simulink model "ARDroneReplay_V2_second"  (R2020a)
settings: Solver=ode1  StartTime=0.0  StopTime=30  FixedStep=sampleTime  RelTol=1e-3  EnableMultiTasking=on
undefined symbols (not defined in the file): Continuous, sampleTime, Time
libraries: ctrlSharedLib x2, ARBlocks x1
settings Model: SimulationMode=accelerator  ExtModeTrigDuration=100000  Creator=Paul  LastModifiedBy=TowerWindows
settings DataIOCC: LimitDataPoints=on  SaveFormat=Array  SignalLoggingSaveFormat=ModelDataLogs  ReturnWorkspaceOutputs=off  TimeSaveName=time
settings OptimizationCC: ExpressionDepthLimit=2147483647  InitFltsAndDblsToZero=on
settings DebuggingCC: UnderspecifiedInitializationDetection=Classic  MergeDetectMultiDrivingBlocksExec=none  SolverPrmCheckMsg=warning  FcnCallInpInsideContextMsg=warning  StateNameClashWarn=warning  SFUnexpectedBacktrackingDiag=warning  SFNoUnconditionalDefaultTransitionDiag=warning  SFExecutionAtInitializationDiag=none  ArithmeticOperatorsInVariantConditions=warning
settings ModelReferenceCC: PropagateSignalLabelsOutOfModel=off
settings SFSimCC: SimUseLocalCustomCode=off  CustomCodeUndefinedFunction=UseInterfaceOnly
settings RTWCC: Description=Simulink Desktop Real-Time  SystemTargetFile=sldrt.tlc  TemplateMakefile=sldrt.tmf  RTWUseLocalCustomCode=off  RTWCompilerOptimization=on
settings CodeAppCC: MaxIdLength=95  StateflowObjectComments=on
settings SimulinkDesktopRealTimeCC: TargetPreCompLibLocation=C:\Program Files\MATLAB\R2020a\toolbox\sldrt\lib\win64  TargetLangStandard=C89/C90 (ANSI)  SupportVariableSizeSignals=off
settings ConfigComp: CovMetricSettings=dw  CovHtmlReporting=on  CovSaveCumulativeToWorkspaceVar=on  CovSaveSingleToWorkspaceVar=on  CovExternalEMLEnable=off

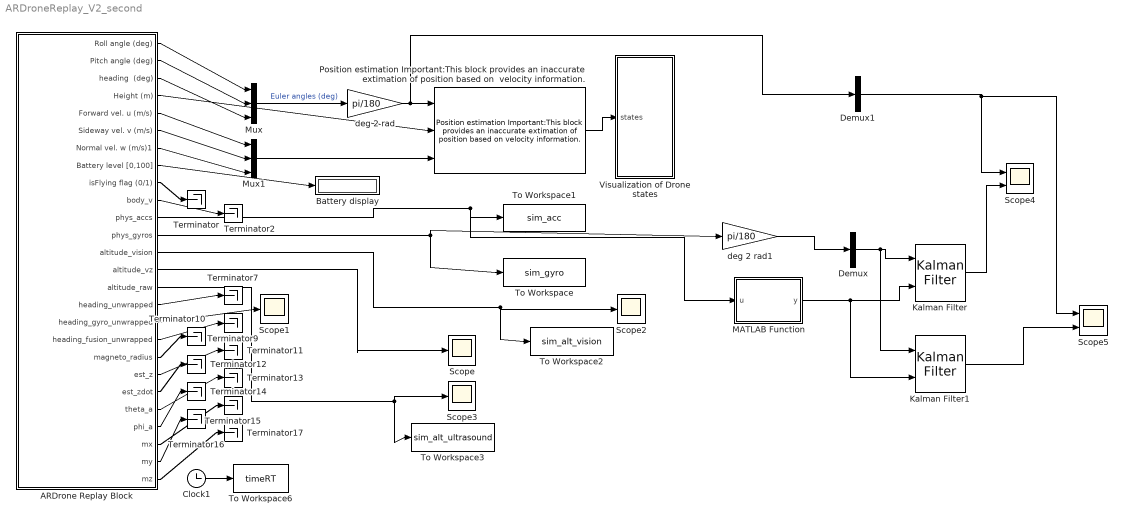
== system ARDroneReplay_V2_second ==
  ARDrone Replay Block : Subsystem  AncestorBlock="ARBlocks/ARDrone Wi-Fi  Block"
  Battery display : Display
  Clock1 : Clock
  Demux : Demux  Outputs=3
  Demux1 : Demux  Outputs=3
  Kalman Filter : ctrlSharedLib/Kalman Filter  TimeDomain=Continuous-Time  UseCurrentEstimator=on  ModelSource=Individual A, B, C, D matrices  ModelSourceVariable=ss(0.95,1,1,0,1)  A=[0 -1; 0 0]  B=[1 ; 0]  C=[1 0]  D=0  NumberOfStates=1  NumberOfInputs=1  NumberOfOutputs=1  InitialEstimateSource=Dialog  X0=0  P0=10  UseK=off  UseGH=off  NumberOfProcessNoiseInputs=1  G=1  TimeInvariantG=on  H=0  TimeInvariantH=on  Q=[0.00081 0; 0 0.0081]  TimeInvariantQ=on  R=25.25  TimeInvariantR=on  N=0  TimeInvariantN=on  AddInputPort=on  AddEnablePort=off  OutputEstimatedY=off  OutputP=off  Ts=-1
  Kalman Filter1 : ctrlSharedLib/Kalman Filter  TimeDomain=Continuous-Time  UseCurrentEstimator=on  ModelSource=Individual A, B, C, D matrices  ModelSourceVariable=ss(0.95,1,1,0,1)  A=0  B=1  C=1  D=0  NumberOfStates=1  NumberOfInputs=1  NumberOfOutputs=1  InitialEstimateSource=Dialog  X0=0  P0=10  UseK=off  UseGH=off  NumberOfProcessNoiseInputs=1  G=1  TimeInvariantG=on  H=0  TimeInvariantH=on  Q=0.00081  TimeInvariantQ=on  R=25.25  TimeInvariantR=on  N=0  TimeInvariantN=on  AddInputPort=on  AddEnablePort=off  OutputEstimatedY=off  OutputP=off  Ts=-1
  MATLAB Function : MATLAB Function  TreatAsAtomicUnit=on
  Mux : Mux  Inputs=3
  Mux1 : Mux  Inputs=3
  "Position estimation Important:This block provides an inaccurate extimation of position based on  velocity information. " : ARBlocks/Position estimation Important:This block provides an  inaccurate extimation of position  based on  velocity information.   SystemSampleTime=-1  Latency=0  AutoFrameSizeCalculation=off
  Scope{,1..3} (4 alike) : Scope
  Scope4 : Scope  NumInputPorts=2
  Scope5 : Scope  NumInputPorts=2
  Terminator{,2,7,9..17} (12 alike) : Terminator
  To Workspace : ToWorkspace  VariableName=sim_gyro  SaveFormat=Timeseries  SampleTime=-1
  To Workspace1 : ToWorkspace  VariableName=sim_acc  SaveFormat=Timeseries  SampleTime=-1
  To Workspace2 : ToWorkspace  VariableName=sim_alt_vision  SaveFormat=Timeseries  SampleTime=-1
  To Workspace3 : ToWorkspace  VariableName=sim_alt_ultrasound  SaveFormat=Timeseries  SampleTime=-1
  To Workspace6 : ToWorkspace  VariableName=timeRT  SampleTime=sampleTime
  Visualization of Drone states : Subsystem
  deg 2 rad : Gain  Gain=pi/180
  deg 2 rad1 : Gain  Gain=pi/180
  wires:
  ARDrone Replay Block/1(Roll angle (deg)) -> Mux/1
  ARDrone Replay Block/2(Pitch angle (deg)) -> Mux/2
  ARDrone Replay Block/5(Forward vel. u (m/s)) -> Mux1/1
  ARDrone Replay Block/6(Sideway vel. v (m/s)) -> Mux1/2
  ARDrone Replay Block/7(Normal vel. w (m/s)1) -> Mux1/3
  Mux/1 -> deg 2 rad/1  "Euler angles (deg)"
  ARDrone Replay Block/8(Battery level [0,100]) -> Battery display/1
  "Position estimation Important:This block provides an inaccurate extimation of position based on  velocity information. "/1 -> Visualization of Drone states/1(states)
  deg 2 rad/1 -> Demux1/1, "Position estimation Important:This block provides an inaccurate extimation of position based on  velocity information. "/1
  ARDrone Replay Block/4(Height (m)) -> "Position estimation Important:This block provides an inaccurate extimation of position based on  velocity information. "/2
  Mux1/1 -> "Position estimation Important:This block provides an inaccurate extimation of position based on  velocity information. "/3
  ARDrone Replay Block/3(heading  (deg)) -> Mux/3
  ARDrone Replay Block/9(isFlying flag (0/1)) -> Terminator/1
  Clock1/1 -> To Workspace6/1
  ARDrone Replay Block/15(altitude_raw) -> To Workspace3/1, Scope3/1
  ARDrone Replay Block/10(body_v) -> Terminator2/1
  ARDrone Replay Block/14(altitude_vz) -> Scope/1
  ARDrone Replay Block/17(heading_gyro_unwrapped) -> Scope1/1
  ARDrone Replay Block/16(heading_unwrapped) -> Terminator7/1
  ARDrone Replay Block/19(magneto_radius) -> Terminator10/1
  ARDrone Replay Block/18(heading_fusion_unwrapped) -> Terminator9/1
  ARDrone Replay Block/21(est_zdot) -> Terminator12/1
  ARDrone Replay Block/20(est_z) -> Terminator11/1
  ARDrone Replay Block/23(phi_a) -> Terminator14/1
  ARDrone Replay Block/22(theta_a) -> Terminator13/1
  ARDrone Replay Block/25(my) -> Terminator16/1
  ARDrone Replay Block/24(mx) -> Terminator15/1
  ARDrone Replay Block/26("mz ") -> Terminator17/1
  ARDrone Replay Block/11(phys_accs) -> MATLAB Function/1(u), To Workspace1/1
  ARDrone Replay Block/13(altitude_vision) -> To Workspace2/1, Scope2/1
  ARDrone Replay Block/12(phys_gyros) -> To Workspace/1, deg 2 rad1/1
  deg 2 rad1/1 -> Demux/1
  Kalman Filter/1 -> Scope4/2
  Demux1/2 -> Scope5/1, Scope4/1
  MATLAB Function/1(y) -> Kalman Filter1/2, Kalman Filter/2
  Demux/2 -> Kalman Filter1/1, Kalman Filter/1
  Kalman Filter1/1 -> Scope5/2

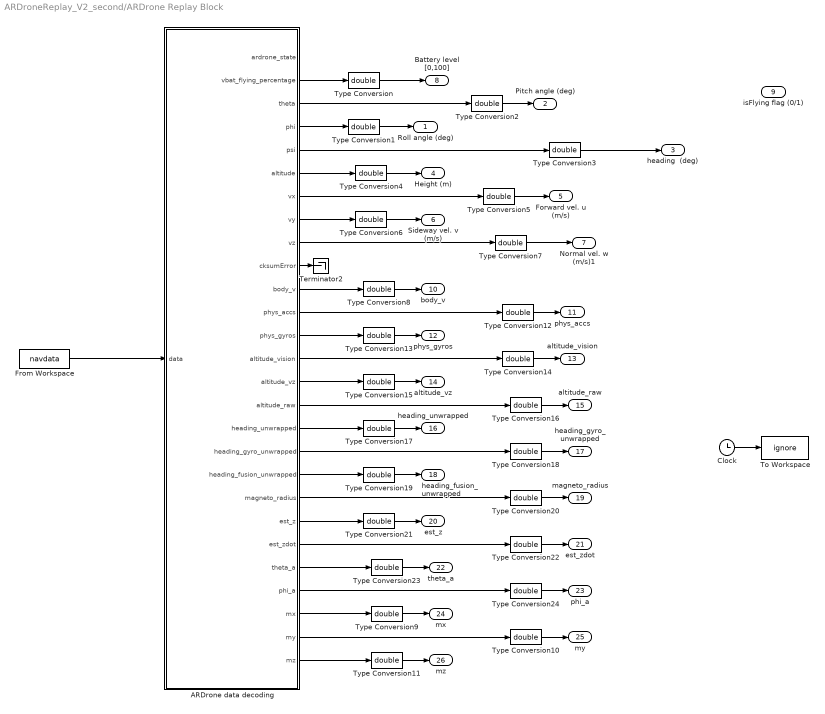
== system ARDroneReplay_V2_second/ARDrone Replay Block ==
  ARDrone data decoding : MATLAB Function  TreatAsAtomicUnit=on
  Clock : Clock
      settings: Decimation=100
  From Workspace : FromWorkspace  VariableName=navdata
  Terminator2 : Terminator
  To Workspace : ToWorkspace  VariableName=ignore  SaveFormat=Timeseries  SampleTime=-1
  Type Conversion{,1..24} (25 alike) : DataTypeConversion  OutDataTypeStr=double
  Roll angle (deg) : Outport  VectorParamsAs1DForOutWhenUnconnected=off
  Pitch angle (deg) : Outport  Port=2  VectorParamsAs1DForOutWhenUnconnected=off
  heading  (deg) : Outport  Port=3  VectorParamsAs1DForOutWhenUnconnected=off
  Height (m) : Outport  Port=4  VectorParamsAs1DForOutWhenUnconnected=off
  Forward vel. u (m/s) : Outport  Port=5  VectorParamsAs1DForOutWhenUnconnected=off
  Sideway vel. v (m/s) : Outport  Port=6  VectorParamsAs1DForOutWhenUnconnected=off
  Normal vel. w (m/s)1 : Outport  Port=7  VectorParamsAs1DForOutWhenUnconnected=off
  Battery level [0,100] : Outport  Port=8  VectorParamsAs1DForOutWhenUnconnected=off
  isFlying flag (0/1) : Outport  Port=9  VectorParamsAs1DForOutWhenUnconnected=off
  body_v : Outport  Port=10  VectorParamsAs1DForOutWhenUnconnected=off
  phys_accs : Outport  Port=11  VectorParamsAs1DForOutWhenUnconnected=off
  phys_gyros : Outport  Port=12  VectorParamsAs1DForOutWhenUnconnected=off
  altitude_vision : Outport  Port=13  VectorParamsAs1DForOutWhenUnconnected=off
  altitude_vz : Outport  Port=14  VectorParamsAs1DForOutWhenUnconnected=off
  altitude_raw : Outport  Port=15  VectorParamsAs1DForOutWhenUnconnected=off
  heading_unwrapped : Outport  Port=16  VectorParamsAs1DForOutWhenUnconnected=off
  heading_gyro_unwrapped : Outport  Port=17  VectorParamsAs1DForOutWhenUnconnected=off
  heading_fusion_unwrapped : Outport  Port=18  VectorParamsAs1DForOutWhenUnconnected=off
  magneto_radius : Outport  Port=19  VectorParamsAs1DForOutWhenUnconnected=off
  est_z : Outport  Port=20  VectorParamsAs1DForOutWhenUnconnected=off
  est_zdot : Outport  Port=21  VectorParamsAs1DForOutWhenUnconnected=off
  theta_a : Outport  Port=22  VectorParamsAs1DForOutWhenUnconnected=off
  phi_a : Outport  Port=23  VectorParamsAs1DForOutWhenUnconnected=off
  mx : Outport  Port=24  VectorParamsAs1DForOutWhenUnconnected=off
  my : Outport  Port=25  VectorParamsAs1DForOutWhenUnconnected=off
  "mz " : Outport  Port=26  VectorParamsAs1DForOutWhenUnconnected=off
  wires:
  Type Conversion/1 -> Battery level [0,100]/1
  Type Conversion1/1 -> Roll angle (deg)/1
  Type Conversion2/1 -> Pitch angle (deg)/1
  Type Conversion4/1 -> Height (m)/1
  Type Conversion5/1 -> Forward vel. u (m/s)/1
  Type Conversion6/1 -> Sideway vel. v (m/s)/1
  Type Conversion7/1 -> Normal vel. w (m/s)1/1
  Type Conversion3/1 -> heading  (deg)/1
  Clock/1 -> To Workspace/1
  Type Conversion8/1 -> body_v/1
  Type Conversion12/1 -> phys_accs/1
  Type Conversion13/1 -> phys_gyros/1
  Type Conversion14/1 -> altitude_vision/1
  Type Conversion15/1 -> altitude_vz/1
  Type Conversion16/1 -> altitude_raw/1
  Type Conversion17/1 -> heading_unwrapped/1
  Type Conversion18/1 -> heading_gyro_unwrapped/1
  Type Conversion19/1 -> heading_fusion_unwrapped/1
  Type Conversion20/1 -> magneto_radius/1
  Type Conversion21/1 -> est_z/1
  Type Conversion22/1 -> est_zdot/1
  Type Conversion23/1 -> theta_a/1
  Type Conversion24/1 -> phi_a/1
  ARDrone data decoding/2(vbat_flying_percentage) -> Type Conversion/1
  ARDrone data decoding/3(theta) -> Type Conversion2/1
  ARDrone data decoding/4(phi) -> Type Conversion1/1
  ARDrone data decoding/5(psi) -> Type Conversion3/1
  ARDrone data decoding/6(altitude) -> Type Conversion4/1
  ARDrone data decoding/7(vx) -> Type Conversion5/1
  ARDrone data decoding/8(vy) -> Type Conversion6/1
  ARDrone data decoding/9(vz) -> Type Conversion7/1
  ARDrone data decoding/10(cksumError) -> Terminator2/1
  ARDrone data decoding/11(body_v) -> Type Conversion8/1
  ARDrone data decoding/12(phys_accs) -> Type Conversion12/1
  ARDrone data decoding/13(phys_gyros) -> Type Conversion13/1
  ARDrone data decoding/14(altitude_vision) -> Type Conversion14/1
  ARDrone data decoding/15(altitude_vz) -> Type Conversion15/1
  ARDrone data decoding/16(altitude_raw) -> Type Conversion16/1
  ARDrone data decoding/17(heading_unwrapped) -> Type Conversion17/1
  ARDrone data decoding/18(heading_gyro_unwrapped) -> Type Conversion18/1
  ARDrone data decoding/19(heading_fusion_unwrapped) -> Type Conversion19/1
  ARDrone data decoding/20(magneto_radius) -> Type Conversion20/1
  ARDrone data decoding/21(est_z) -> Type Conversion21/1
  ARDrone data decoding/22(est_zdot) -> Type Conversion22/1
  ARDrone data decoding/23(theta_a) -> Type Conversion23/1
  ARDrone data decoding/24(phi_a) -> Type Conversion24/1
  Type Conversion9/1 -> mx/1
  ARDrone data decoding/25(mx) -> Type Conversion9/1
  Type Conversion10/1 -> my/1
  ARDrone data decoding/26(my) -> Type Conversion10/1
  Type Conversion11/1 -> "mz "/1
  ARDrone data decoding/27(mz) -> Type Conversion11/1
  From Workspace/1 -> ARDrone data decoding/1(data)

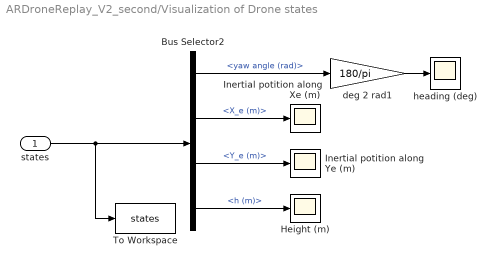
== system ARDroneReplay_V2_second/Visualization of Drone states ==
  states : Inport
  Bus Selector2 : BusSelector  OutputSignals=yaw angle (rad),X_e (m),Y_e (m),h (m)
  Height (m) : Scope
  Inertial potition along Xe (m) : Scope
  Inertial potition along Ye (m) : Scope
  To Workspace : ToWorkspace  VariableName=states  SaveFormat=Structure With Time  SampleTime=-1
  deg 2 rad1 : Gain  Gain=180/pi
  heading (deg) : Scope
  wires:
  states/1 -> To Workspace/1, Bus Selector2/1
  Bus Selector2/1 -> deg 2 rad1/1  "<yaw angle (rad)>"
  Bus Selector2/2 -> Inertial potition along Xe (m)/1  "<X_e (m)>"
  Bus Selector2/3 -> Inertial potition along Ye (m)/1  "<Y_e (m)>"
  Bus Selector2/4 -> Height (m)/1  "<h (m)>"
  deg 2 rad1/1 -> heading (deg)/1

== matlab function ARDroneReplay_V2_second/ARDrone Replay Block/ARDrone data decoding ==
  data: ardrone_state output; vbat_flying_percentage output; theta output; phi output; psi output; altitude output; vx output; vy output; vz output; cksumError output; body_v output; phys_accs output; phys_gyros output; altitude_vision output; altitude_vz output; altitude_raw output; heading_unwrapped output; heading_gyro_unwrapped output; heading_fusion_unwrapped output; magneto_radius output; est_z output; est_zdot output; theta_a output; phi_a output; mx output; my output; data input; mz output
function [ardrone_state, vbat_flying_percentage,...
    theta, phi, psi, altitude, vx, vy, vz , cksumError, body_v,...
    phys_accs,phys_gyros,altitude_vision,altitude_vz,altitude_raw,heading_unwrapped,heading_gyro_unwrapped,...
    heading_fusion_unwrapped,magneto_radius,est_z,est_zdot,theta_a,phi_a,mx, my, mz]= trata_dados_large(data)

%initialize arrays
vbat_flying_percentage = 0;
phi = 0;
theta = 0;
psi = 0;
altitude = 0;
vx = 0;
vy = 0;
vz = 0;
phys_accs=zeros(3,1);
phys_gyros=zeros(3,1);
body_v=zeros(3,1);
theta_a = 0;
phi_a = 0;
altitude_vision = 0; 
altitude_vz = 0;
altitude_raw = 0;
heading_unwrapped=0;
heading_gyro_unwrapped = 0;
heading_fusion_unwrapped = 0;
magneto_radius = 0;
est_z = 0;
est_zdot = 0;
theta_a = 0;
phi_a = 0;
mx = 0;
my = 0; 
mz = 0;

% Checksum array. cksum(1) contains the computed checksum, cksum(2)
% contains the checksum sent by the ARDrone. 
cksum = [0 0]; 

% Computing checksum
cksum(1) =  sum(double(data(1:end-8)))+442; 
% Checksum given by the drone
cksum(2) = double(data(end-3)) + double(data(end-2))*256 +  double(data(end-1))*256^2 + double(data(end))*256^3 ; 
% Checksum error
cksumError = abs(cksum(1)-cksum(2));

% Converting bytes to drone information

% header data
ardrone_state = getDroneState(data(1:4));

% demo data
vbat_flying_percentage(1) = decode_32bit(data(21:24),1); % unit: percentage 0 -100
theta(1) = decode_32bit(data(25:28),0)/1000; % unit: deg
phi(1) = decode_32bit(data(29:32),0)/1000; % unit: deg
psi(1) = decode_32bit(data(33:36),0)/1000; % unit: deg
altitude(1) = decode_32bit(data(37:40),1)/1000; % unit: m
vx(1) = decode_32bit(data(41:44),0)/1000; % unit: m/s
vy(1) = decode_32bit(data(45:48),0)/1000; % unit: m/s
vz(1) = decode_32bit(data(49:52),0)/1000; % unit: m/s
%detection_camera_type(1) = decode_32bit(data(109:112),1);

phys_accs(1) = decode_32bit(data(231:234),0);
phys_accs(2) = decode_32bit(data(235:238),0);
phys_accs(3) = decode_32bit(data(239:242),0);
phys_gyros(1) = decode_32bit(data(243:246),0);
phys_gyros(2) = decode_32bit(data(247:250),0);
phys_gyros(3) = decode_32bit(data(251:254),0);
if (phys_gyros(3)>100)
    phys_gyros(3)=100;
elseif (phys_gyros(3)<-100)
    phys_gyros(3)=-100;
end

% euler angles
theta_a(1) = decode_32bit(data(287:290),0);
phi_a(1) = decode_32bit(data(291:294),0);

altitude_vision(1) = decode_32bit(data(519:522),0);    %%%% typecast(data(519:522), 'int32');
altitude_vz(1) = decode_32bit(data(523:526),0);
altitude_raw(1) = decode_32bit(data(531:534),0);       %%%% typecast(data(531:534), 'int32');
 
heading_unwrapped(1) = decode_32bit(data(1712:1715),0);
heading_gyro_unwrapped(1) = decode_32bit(data(1716:1719),0);
heading_fusion_unwrapped(1) = decode_32bit(data(1720:1723),0);

magneto_radius(1) = decode_32bit(data(1737:1740),0);
% magneto
mx(1) = decode_16bit(data(1670:1671),1);
my(1) = decode_16bit(data(1672:1673),1);
mz(1) = decode_16bit(data(1674:1675),1);

est_z(1) = decode_32bit(data(1821:1824),0);
est_zdot(1) = decode_32bit(data(1825:1828),0);

%cks
%cks = decode_32bit(data(end-3:end),1); 
    
end


function res = decode_32bit(input, mark)
% if mark = 1; then output a int
% else output the float value which is defined by SDK description.
% the input is an array (1*4)
% e.g. : NDS(Battery_OS:Battery_OS+data_length-1)

% hex_value = dec2hex(input);
% hex_value = [hex_value(4,:),hex_value(3,:),hex_value(2,:),hex_value(1,:)];
if mark ==1
    res = typecast(input,'uint32');%hex2dec(hex_value);
elseif mark ==2
    res = hex2dec(hex_value)-2^31;
else
    res = typecast(input,'single');%typecast(uint32(hex2dec(hex_value)),'single');
end
end

function res = decode_16bit(input,mark)
%hex_value = dec2hex(input);
%hex_value = [hex_value(2,:),hex_value(1,:)];
%res = hex2dec(hex_value);
res = typecast(input,'uint16')-2^15;
if mark==1
    res=res-2^15;
end
end

function bin = getDroneState(input)
bin = zeros(32,1);
hex = dec2hex(input);
% put the hex_value in the order [31, 30......0]
hex = [hex(4,:),hex(3,:),hex(2,:),hex(1,:)];
for i=1:length(hex)
    if hex(i)=='F'
        bin((i*4)-3:i*4)=[1 1 1 1];
    elseif hex(i)=='E'
        bin((i*4)-3:i*4)=[1 1 1 0];
    elseif hex(i)=='D'
        bin((i*4)-3:i*4)=[1 1 0 1];
    elseif hex(i)=='C'
        bin((i*4)-3:i*4)=[1 1 0 0];
    elseif hex(i)=='B'
        bin((i*4)-3:i*4)=[1 0 1 1];
    elseif hex(i)=='A'
        bin((i*4)-3:i*4)=[1 0 1 0];
    elseif hex(i)=='9'
        bin((i*4)-3:i*4)=[1 0 0 1];
    elseif hex(i)=='8'
        bin((i*4)-3:i*4)=[1 0 0 0];
    elseif hex(i)=='7'
        bin((i*4)-3:i*4)=[0 1 1 1];
    elseif hex(i)=='6'
        bin((i*4)-3:i*4)=[0 1 1 0];
    elseif hex(i)=='5'
        bin((i*4)-3:i*4)=[0 1 0 1];
    elseif hex(i)=='4'
        bin((i*4)-3:i*4)=[0 1 0 0];
    elseif hex(i)=='3'
        bin((i*4)-3:i*4)=[0 0 1 1];
    elseif hex(i)=='2'
        bin((i*4)-3:i*4)=[0 0 1 0];
    elseif hex(i)=='1'
        bin((i*4)-3:i*4)=[0 0 0 1];
    elseif hex(i)=='0'
        bin((i*4)-3:i*4)=[0 0 0 0];
    end
end

end

== matlab function ARDroneReplay_V2_second/MATLAB Function ==
  data: u input; y output
function y = fcn(u)

y = atan2(u(1)*100,sqrt(((u(3)^2)*100)+((u(2)^2*100))));
